simulink model "Crossovers"  (R2016b)
settings: Solver=VariableStepAuto  StartTime=0.0  StopTime=10.0  RelTol=1e-3
values from neighbouring files (symbols this model uses):
  Fs = 48000    [Coefficient_Calculator.m]    (also in Coefficient_Calculator_2.m; Initializiation.m; Time_varying_BP.m)
libraries: dspsrcs4 x1
settings Model: Creator=Bagas Prabowo  LastModifiedBy=Bagas Prabowo

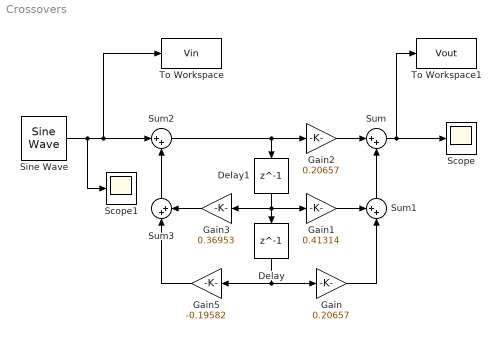
== system Crossovers ==
  Delay : Delay  DelayLength=1
  Delay1 : Delay  DelayLength=1
  Gain : Gain  Gain=0.20657
  Gain1 : Gain  Gain=0.41314
  Gain2 : Gain  Gain=0.20657
  Gain3 : Gain  Gain=0.36953
  Gain5 : Gain  Gain=-0.19582
  Scope : Scope
  Scope1 : Scope
  Sine Wave : dspsrcs4/Sine Wave  Amplitude=1  Frequency=5000  Phase=0  SampleMode=Discrete  OutComplex=Real  CompMethod=Trigonometric fcn  TableSize=Speed  SampleTime=1/Fs  SamplesPerFrame=1  ResetState=Restart at time zero  OutputFrames=off  dataType=double  wordLen=16  udDataType=sfix(16)  fracBitsMode=Best precision  numFracBits=15  OutDataTypeStr=double  LastOutDataTypeStr=double
  Sum : Sum  Inputs=|++
  Sum1 : Sum  Inputs=++|
  Sum2 : Sum  Inputs=|++
  Sum3 : Sum  Inputs=|++
  To Workspace : ToWorkspace  VariableName=Vin  SampleTime=-1
      settings: Save2DSignal=2-D array (concatenate along first dimension)
  To Workspace1 : ToWorkspace  VariableName=Vout  SampleTime=-1
      settings: Save2DSignal=2-D array (concatenate along first dimension)
  wires:
  Delay/1 -> Gain/1, Gain5/1
  Gain1/1 -> Sum1/1
  Gain/1 -> Sum1/2
  Sum1/1 -> Sum/2
  Gain2/1 -> Sum/1
  Delay1/1 -> Gain3/1, Gain1/1, Delay/1
  Gain3/1 -> Sum3/2
  Gain5/1 -> Sum3/1
  Sum3/1 -> Sum2/2
  Sum2/1 -> Gain2/1, Delay1/1
  Sum/1 -> To Workspace1/1, Scope/1
  Sine Wave/1 -> Scope1/1, To Workspace/1, Sum2/1
